simulink model "flight_dynamics"  (R2016b)
settings: Solver=FixedStepAuto  StartTime=0.0  StopTime=10000  FixedStep=.005  RelTol=1e-3  EnableMultiTasking=on
InitFcn:
  | param
undefined symbols (not defined in the file or in its folder): drawAircraft, forces_moments, P, plotmavstatevariables
libraries: dspsrcs4 x1
settings Model: Creator=nmd89  LastModifiedBy=nmd89
settings OptimizationCC: LifeSpan=inf
settings DebuggingCC: SFUnexpectedBacktrackingDiag=warning  SFNoUnconditionalDefaultTransitionDiag=warning  SFExecutionAtInitializationDiag=none
settings GRTTargetCC: TargetLangStandard=C89/C90 (ANSI)  GeneratePreprocessorConditionals=Disable all
settings ConfigComp: CovMetricSettings=dw  CovHtmlReporting=on  CovSaveCumulativeToWorkspaceVar=on  CovSaveSingleToWorkspaceVar=on  CovExternalEMLEnable=off

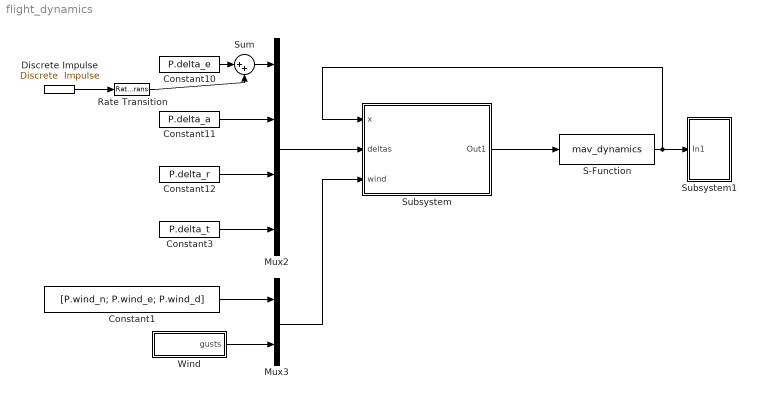
== system flight_dynamics ==
  Constant1 : Constant  Value=[P.wind_n; P.wind_e; P.wind_d]
  Constant10 : Constant  Value=P.delta_e
  Constant11 : Constant  Value=P.delta_a
  Constant12 : Constant  Value=P.delta_r
  Constant3 : Constant  Value=P.delta_t
  Discrete Impulse : dspsrcs4/Discrete  Impulse  Delay=5  SampleTime=0.1  FrameSample=1  OutputFrames=off  dataType=double  isSigned=on  wordLen=16  udDataType=sfix(16)  fracBitsMode=Best precision  numFracBits=15  OutDataTypeStr=double  LastOutDataTypeStr=double
  Mux2 : Mux
  Mux3 : Mux  Inputs=2
  Rate Transition : RateTransition
  S-Function : S-Function  FunctionName=mav_dynamics  Parameters=P  SFunctionDeploymentMode=off  EnableBusSupport=off
  Subsystem : Subsystem
  Subsystem1 : Subsystem
  Sum : Sum  Inputs=|++
  Wind : Subsystem
  wires:
  S-Function/1 -> Subsystem1/1(In1), Subsystem/1("x ")
  Wind/1(gusts) -> Mux3/2
  Constant1/1 -> Mux3/1
  Constant3/1 -> Mux2/4
  Subsystem/1(Out1) -> S-Function/1
  Mux2/1 -> Subsystem/2(deltas)
  Mux3/1 -> Subsystem/3(wind)
  Discrete Impulse/1 -> Rate Transition/1
  Rate Transition/1 -> Sum/2
  Constant11/1 -> Mux2/2
  Constant12/1 -> Mux2/3
  Constant10/1 -> Sum/1
  Sum/1 -> Mux2/1

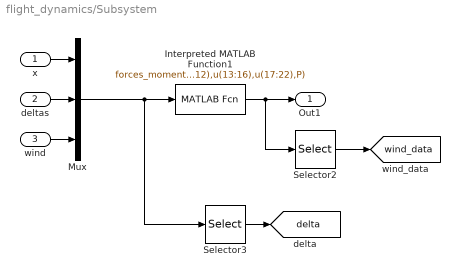
== system flight_dynamics/Subsystem ==
  "x " : Inport
  deltas : Inport  Port=2
  wind : Inport  Port=3
  Interpreted MATLAB Function1 : MATLABFcn  MATLABFcn=forces_moments(u(1:12),u(13:16),u(17:22),P)
  Mux : Mux  Inputs=3
  Selector2 : Selector  InputPortWidth=12  IndexOptions=Index vector (dialog)  Indices=[7 8 9 10 11 12]  OutputSizes=1
  Selector3 : Selector  InputPortWidth=22  IndexOptions=Index vector (dialog)  Indices=[13 14 15 16]  OutputSizes=1
  Out1 : Outport
  tag scope: delta=global, wind_data=global
  wires:
  Mux/1 -> Selector3/1, Interpreted MATLAB Function1/1
  Interpreted MATLAB Function1/1 -> Selector2/1, Out1/1
  "x "/1 -> Mux/1
  deltas/1 -> Mux/2
  wind/1 -> Mux/3
  Selector2/1 -> [wind_data]
  Selector3/1 -> [delta]

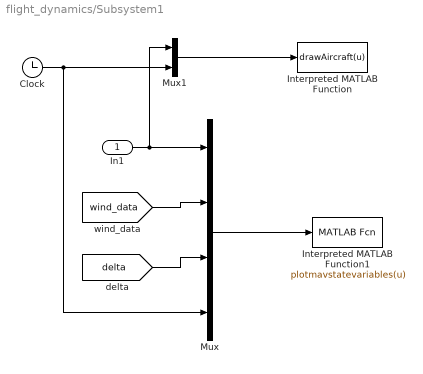
== system flight_dynamics/Subsystem1 ==
  In1 : Inport
  Clock : Clock
  Interpreted MATLAB Function : MATLABFcn  MATLABFcn=drawAircraft(u)  OutputDimensions=0
  Interpreted MATLAB Function1 : MATLABFcn  MATLABFcn=plotmavstatevariables(u)  OutputDimensions=0
  Mux : Mux
  Mux1 : Mux  Inputs=2
  wires:
  In1/1 -> Mux1/1, Mux/1
  Mux/1 -> Interpreted MATLAB Function1/1
  [wind_data] -> Mux/2
  [delta] -> Mux/3
  Mux1/1 -> Interpreted MATLAB Function/1
  Clock/1 -> Mux1/2, Mux/4

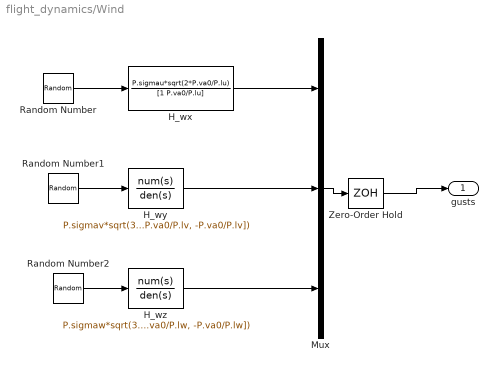
== system flight_dynamics/Wind ==
  H_wx : TransferFcn  Numerator=P.sigmau*sqrt(2*P.va0/P.lu)  Denominator=[1 P.va0/P.lu]
  H_wy : TransferFcn  Numerator=P.sigmav*sqrt(3*P.va0/P.lv)*[0, 1, P.va0/sqrt(3)/P.lv]  Denominator=poly([-P.va0/P.lv, -P.va0/P.lv])
  H_wz : TransferFcn  Numerator=P.sigmaw*sqrt(3*P.va0/P.lw)*[0, 1, P.va0/sqrt(3)/P.lw]  Denominator=poly([-P.va0/P.lw, -P.va0/P.lw])
  Mux : Mux  Inputs=3
  Random Number : RandomNumber  SampleTime=0
  Random Number1 : RandomNumber  SampleTime=0
  Random Number2 : RandomNumber  SampleTime=0
  Zero-Order Hold : ZeroOrderHold  SampleTime=P.Ts
  gusts : Outport
  wires:
  H_wx/1 -> Mux/1
  Random Number/1 -> H_wx/1
  H_wy/1 -> Mux/2
  Random Number1/1 -> H_wy/1
  H_wz/1 -> Mux/3
  Random Number2/1 -> H_wz/1
  Mux/1 -> Zero-Order Hold/1
  Zero-Order Hold/1 -> gusts/1
